simulink model "Racing_2019"  (R2017a)
settings: Solver=FixedStepDiscrete  StartTime=0.0  StopTime=Inf  FixedStep=1e-3  RelTol=1e-3  EnableMultiTasking=on
PostLoadFcn:
  | , if any(exist('dsrtsu_mdlpostloadfcn', 'file') == [2, 3, 6]), try dsrtsu_mdlpostloadfcn('Execute', bdroot); catch fprintf('Error in PostLoadFcn (dsrtsu_mdlpostloadfcn) for model "%s":\n %s\n', bdroot, lasterr); end, end,
undefined symbols (not defined in the file): Accu_Fans_Enable, Accu_Fans_ON, Accu_Fans_PWM, APPS_Bypass, APPS_Value, AUX_Error_Time, Batt_Temp_High_Threshold, Batt_Temp_Low_Threshold, BMS_Error_Time, BMS_Reset, BMS_Reset_Enable, BMS_Status_Bypass, Brake_Plausibility_Threshold, Brake_Threshold, Brakelight_Test, Braking_Torque, BSPD_State_Bypass, Buzzer, Buzzer_Silent, Buzzer_Test, Calibrate, CAN_Rx_FMEA_Enable, CAN_Status_FMEA_Enable, CAN_Tx_FMEA_Enable, Car_Reset, Car_Reset_Enable, Dash_Fan_PWM, DiscIntNeverNeededParam, DRS_Enable, DRS_PWM_OFF, DRS_PWM_ON, ED_Enable, ED_On, Eject_USB, Enable_Kill, Enable_LED_Test, Fans_Left_Enable, Fans_Left_ON, Fans_Left_PWM, Fans_Right_Enable, Fans_Right_ON, Fans_Right_PWM, I_MAX, IGBT_Temp_High_Threshold, IGBT_Temp_Low_Threshold, Inverter_CAN_Tx_Enable, Inverter_Frequency, KW_Max_Regen_Reset, KW_Max_Reset, LV_DCDC_Temp_High_Threshold, LV_DCDC_Temp_Low_Threshold, magnitude, Plausibility_Bypass, Power_Limiter_Killswitch, Power_Target_kW, Pump_Left_Enable, Pump_Left_ON, Pump_Right_Enable, Pump_Right_ON, Pump_Signal_Left ... (+13)
libraries: rtiusbflightreclib x206, simulink x153, rtican x52, powerlib_meascontrol x47, simulink_extras x17, rti1401lib_adc_type4 x6, rti1401lib_dio_type4 x3, rti1401lib_II_base x1
(part 1 of 23)
PreSaveFcn:
  | , if any(exist('dsmpb_private', 'file') == [2, 3, 6]), try, dsmpb_private('dsmpb_mdlclblib', 'PreSave', bdroot); catch, disp(lasterr); end, end,
CloseFcn:
  | , if any(exist('dsmpb_private', 'file') == [2, 3, 6]), try, dsmpb_private('dsmpb_mdlclblib', 'Close', bdroot); catch, disp(lasterr); end, end,
Description:
  | Standard RTI1401 template.
  | Supported Matlab version:  R2017a.
settings Model: Tag=RTI1401  DSRTSU_INTERNAL_RTI_VER=500  DSRTSU_INTERNAL_RTI_TYPE=rti1401  RTICANMMDATA=struct('GeneralSetupData',struct('modelroot',['C:\Users\Vasileios Amoiridis\Documents\dSpaceProjects\R2017a_Racing_2019'],'generalsettings',struct('filesettings',struct('destfolder',struct('Name','RTICANMM_FILES','Check',1),'buildfolder',struct('Name','.','Check',1),'AbsDestfolder',struct('Name',['C:\Users\Vasileios Amoiridis\Documents\dSpaceProjects\R2017a_Racing_2019\RTICANMM_FILES']),'AbsBuildfolder',struct('Name',['C:\Users\Vasileios Amoiridis\Documents\dSpaceProjects\R2017a_Racing_2019']))),'options',struct('addpaths',1,'rmpaths',1,'addtrcexclusion',logical(1),'cannavigator',struct('checkmonitoring',0),'show_usrtrc',0,'use_usrtrc',0),'advanced',struct('options',ones(1,100)),'MPSetup',{{}},'modelname','Racing_2019','block','Racing_2019'))  DSRTSU_INTERNAL_RTIFPGA=90  DSMPB_DATASERVER_ModelPortLibVersion1=8  DSMPB_DATASERVER_DataServerVersion1=6  DSMPB_DATASERVER_DataServerStreamVersion1=3  Creator=Vasileios Amoiridis  LastModifiedBy=Vasileios Amoiridis
settings DataIOCC: SaveOutput=off  SignalLogging=off  DSMLogging=off  SaveTime=off
settings OptimizationCC: BlockReduction=off  ConditionallyExecuteInputs=off  OptimizeBlockIOStorage=off  BufferReuse=off  GlobalBufferReuse=off  ExpressionFolding=off  LocalBlockOutputs=off  LifeSpan=inf
settings DebuggingCC: SFUnexpectedBacktrackingDiag=warning  SFNoUnconditionalDefaultTransitionDiag=warning  SFExecutionAtInitializationDiag=none
settings HardwareCC: ProdBitPerPointer=32  ProdBitPerSizeT=32  ProdBitPerPtrDiffT=32  ProdLargestAtomicInteger=Integer  ProdEndianess=BigEndian  ProdWordSize=32  ProdHWDeviceType=Custom Processor->Custom  TargetIntDivRoundTo=Zero  TargetEndianess=BigEndian  TargetHWDeviceType=Custom Processor->Custom
settings SFSimCC: MATLABDynamicMemAlloc=off
settings RTWCC: SystemTargetFile=rti1401.tlc  MakeCommand=make_rti  TemplateMakefile=rti1401.tmf  Description=dSPACE DS1401 Hardware Platform
settings CodeAppCC: GenerateComments=off  SimulinkBlockComments=off
settings STFCustomTargetCC: ParMdlRefBuildCompliant=on  GRTInterface=off  SystemTargetFile=rti1401.tlc
settings GRTTargetCC: TargetLangStandard=C89/C90 (ANSI)  CompOptLevelCompliant=off  ConcurrentExecutionCompliant=off  CombineOutputUpdateFcns=off  MatFileLogging=off  CPPClassGenCompliant=off  UseToolchainInfoCompliant=off
settings ConfigComp: CovMetricSettings=dswe  CovSaveCumulativeToWorkspaceVar=on

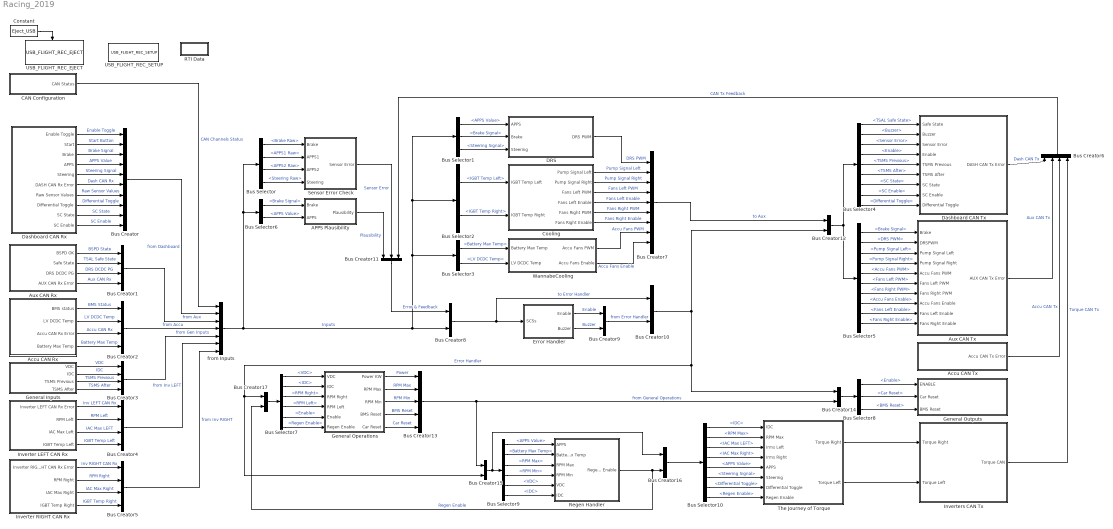
== system Racing_2019 ==
  APPS Plausibility : Subsystem
  Accu CAN Rx : Subsystem
  Accu CAN Tx : Subsystem
  Aux CAN Rx : Subsystem
  Aux CAN Tx : Subsystem
  Bus Creator : BusCreator  Inputs='Enable Toggle','Start Button','Brake Signal','APPS Value','Steering Signal','Dash CAN Rx','Raw Sensor Values','Differential Toggle','SC State','SC Enable'
  Bus Creator1 : BusCreator  Inputs='BSPD State','TSAL Safe State','DRS DCDC PG','Aux CAN Rx'
  Bus Creator{10,12,14..16} (5 alike) : BusCreator  Inputs=2
  Bus Creator11 : BusCreator  Inputs=3
  Bus Creator13 : BusCreator  Inputs=5
  Bus Creator17 : BusCreator  Inputs='Error Handler','Regen Enable'
  Bus Creator2 : BusCreator  Inputs='BMS Status','LV DCDC Temp','Accu CAN Rx','Battery Max Temp'
  Bus Creator3 : BusCreator  Inputs='VDC','IDC','TSMS Previous','TSMS After'
  Bus Creator4 : BusCreator  Inputs='Inv LEFT CAN Rx','RPM Left','IAC Max LEFT','IGBT Temp Left'
  Bus Creator5 : BusCreator  Inputs='Inv RIGHT CAN Rx','RPM Right','IAC Max Right','IGBT Temp Right'
  Bus Creator6 : BusCreator  Inputs='Dash CAN Tx','Aux CAN Tx','Accu CAN Tx','Torque CAN Tx'
  Bus Creator7 : BusCreator  Inputs='DRS PWM','Pump Signal Left','Pump Signal Right','Fans Left PWM','Fans Left Enable','Fans Right PWM','Fans Right Enable','Accu Fans PWM','Accu Fans Enable'
  Bus Creator8 : BusCreator  Inputs='Error & Feedback','Inputs'
  Bus Creator9 : BusCreator  Inputs='Enable','Buzzer'
  Bus Selector : BusSelector  OutputSignals=from Dashboard.Raw Sensor Values.Brake Raw,from Dashboard.Raw Sensor Values.APPS1 Raw,from Dashboard.Raw Sensor Values.APPS2 Raw,from Dashboard.Raw Sensor Values.Steering Raw
  Bus Selector1 : BusSelector  OutputSignals=from Dashboard.APPS Value,from Dashboard.Brake Signal,from Dashboard.Steering Signal
  Bus Selector10 : BusSelector  OutputSignals=signal1.Error Handler.to Error Handler.Inputs.from Gen Inputs.IDC,signal1.from General Operations.RPM Max,signal1.Error Handler.to Error Handler.Inputs.from Inv LEFT.IAC Max LEFT,signal1.Error Handler.to Error Handler.Inputs.from Inv RIGHT.IAC Max Right,signal1.Error Handler.to Error Handler.Inputs.from Dashboard.APPS Value,signal1.Error Handler.to Error Handler.Inputs.from Dashboard.Steering Signal,signal1.Error Handler.to Error Handler.Inputs.from Dashboard.Differential Toggle,Regen Enable
  Bus Selector2 : BusSelector  OutputSignals=from Inv LEFT.IGBT Temp Left,from Inv RIGHT.IGBT Temp Right
  Bus Selector3 : BusSelector  OutputSignals=from Accu.Battery Max Temp,from Accu.LV DCDC Temp
  Bus Selector4 : BusSelector  OutputSignals=Error Handler.to Error Handler.Inputs.from Aux.TSAL Safe State,Error Handler.from Error Handler.Buzzer,Error Handler.to Error Handler.Error & Feedback.Sensor Error,Error Handler.from Error Handler.Enable,Error Handler.to Error Handler.Inputs.from Gen Inputs.TSMS Previous,Error Handler.to Error Handler.Inputs.from Gen Inputs.TSMS After,Error Handler.to Error Handler.Inputs.from Dashboard.SC State,Error Handler.to Error Handler.Inputs.from Dashboard.SC Enable,Error Handler.to Error Handler.Inputs.from Dashboard.Differential Toggle
  Bus Selector5 : BusSelector  OutputSignals=Error Handler.to Error Handler.Inputs.from Dashboard.Brake Signal,to Aux.DRS PWM,to Aux.Pump Signal Left,to Aux.Pump Signal Right,to Aux.Accu Fans PWM,to Aux.Fans Left PWM,to Aux.Fans Right PWM,to Aux.Accu Fans Enable,to Aux.Fans Left Enable,to Aux.Fans Right Enable
  Bus Selector6 : BusSelector  OutputSignals=from Dashboard.Brake Signal,from Dashboard.APPS Value
  Bus Selector7 : BusSelector  OutputSignals=Error Handler.to Error Handler.Inputs.from Gen Inputs.VDC,Error Handler.to Error Handler.Inputs.from Gen Inputs.IDC,Error Handler.to Error Handler.Inputs.from Inv RIGHT.RPM Right,Error Handler.to Error Handler.Inputs.from Inv LEFT.RPM Left,Error Handler.from Error Handler.Enable,Regen Enable
  Bus Selector8 : BusSelector  OutputSignals=Error Handler.from Error Handler.Enable,from General Operations.Car Reset,from General Operations.BMS Reset
  Bus Selector9 : BusSelector  OutputSignals=Error Handler.to Error Handler.Inputs.from Dashboard.APPS Value,Error Handler.to Error Handler.Inputs.from Accu.Battery Max Temp,from General Operations.RPM Max,from General Operations.RPM Min,Error Handler.to Error Handler.Inputs.from Gen Inputs.VDC,Error Handler.to Error Handler.Inputs.from Gen Inputs.IDC
  CAN Configuration : Subsystem
  Constant : Constant  Value=Eject_USB
  Cooling : Subsystem
  DRS : Subsystem
  Dashboard CAN Rx : Subsystem
  Dashboard CAN Tx : Subsystem
  Error Handler : Subsystem
  General Inputs : Subsystem
  General Operations : Subsystem
  "General Outputs " : Subsystem
  Inverter LEFT CAN Rx : Subsystem
  Inverter RIGHT CAN Rx : Subsystem
  Inverters CAN Tx : Subsystem
  RTI Data : Subsystem  Tag=struct('RTIDataServer',struct('RTIDataServerVs','2','RTIModelDescription','struct(''main'',''Racing_2019'',''sub'','''',''isMp'',0)'))  LoadFcn="if exist('rtidc'), try,  rtidc('DataHostBlockClbLoad', gcbh); catch, disp(['Warning: ''LoadFcn'' for RTI Data block failed: ' lasterr]); end, end,"  mask(RTI_DATA_HOST){}
      mask help:
      | RTI Data Block.
      | This block is used by RTI to store internal model-dependent data.
      | Please keep this block on the root level of the model. Deleting this block will result in data loss.
      |
      | NEVER DELETE OR COPY THIS BLOCK!
      settings: CopyFcn="if exist('rtidc'), try,  rtidc('DataHostBlockClbCopy', gcbh); catch, disp(['Warning: ''CopyFcn'' for RTI Data block failed: ' lasterr]); end, end,"  DeleteFcn="if exist('rtidc'), try,  rtidc('DataHostBlockClbDelete', gcbh); catch, disp(['Warning: ''DeleteFcn'' for RTI Data block failed: ' lasterr]); end, end,"  ModelCloseFcn="if exist('rtidc'), try,  rtidc('DataHostBlockClbModelClose', gcbh); catch, disp(['Warning: ''ModelCloseFcn'' for RTI Data block failed: ' lasterr]); end, end,"  PreSaveFcn="if exist('rtidc'), try,  rtidc('DataHostBlockClbPreSave', gcbh); catch, disp(['Warning: ''PreSaveFcn'' for RTI Data block failed: ' lasterr]); end, end,"  PostSaveFcn="if exist('rtidc'), try,  rtidc('DataHostBlockClbPostSave', gcbh); catch, disp(['Warning: ''PostSaveFcn'' for RTI Data block failed: ' lasterr]); end, end,"  NameChangeFcn="if exist('rtidc'), try,  rtidc('DataHostBlockClbNameChange', gcbh); catch, disp(['Warning: ''NameChangeFcn'' for RTI Data block failed: ' lasterr]); end, end,"
      mask Help:
      | RTI Data Block.
      | This block is used by RTI to store internal model-dependent data.
      | Please keep this block on the root level of the model. Deleting this block will result in data loss.
      | 
      | NEVER DELETE OR COPY THIS BLOCK!
      mask Display:
      | text(0.5, 0.5, 'RTI Data', 'HorizontalAlignment', 'center');
      | plot([1 0]);
  Regen Handler : Subsystem
  Sensor Error Check : Subsystem
  The Journey of Torque : Subsystem
  USB_FLIGHT_REC_EJECT : rtiusbflightreclib/USB_FLIGHT_REC_EJECT  DSProperties=struct('RTI',struct('Version',uint32(1),'BlockType',struct('isSLSource',uint8(0),'isSLSink',uint8(1),'isHWSource',uint8(0),'isHWSink',uint8(1),'isSetup',uint8(0),'isInline',uint8(1),'isNonInline',uint8(0),'isInterrupt',uint8(0),'isChannelwise',uint8(1)),'IOBoardType',{{'DSUSB','FLIGHTREC'}},'UnitType','FLIGHTREC','Identifier','EJECT','DialogType','ML','BlockSet','RTIUSBFLIGHTREC','SlaveProcessor','NONE'))  RTIBlockInterface=struct('OutputPortsWidth',int32(1),'OutputPortsActive',0,'TriggerPort',{{'rising'}},'BlockDisplay',{{['USB Flight Recorder\n Eject USB Device'],'center'}},'IconTransparency','on','InitLevel',3,'DialogFcn','rtiusbflightrecejectgui','BlockName',struct('Token',{{'USB_FLIGHT_REC_EJECT'}}))  RTIBlockParameters=struct('TLCFileName',{{'rtiusbflightreceject','OFF',[]}})  RTISFcnParameters=struct('TLCFileName','char')  RTIBlockParaDefault=struct('TLCFileName','rtiusbflightreceject')
      settings: SourceProductName=dSPACE RTI USB Flight Rec Blockset
  USB_FLIGHT_REC_SETUP : rtiusbflightreclib/USB_FLIGHT_REC_SETUP  BufferOverwriteMode=Replace old data  TLCFileName=rtiusbflightrecsetup  DSProperties=struct('RTI',struct('Version',uint32(1),'BlockType',struct('isSLSource',uint8(0),'isSLSink',uint8(0),'isHWSource',uint8(0),'isHWSink',uint8(0),'isSetup',uint8(1),'isInline',uint8(1),'isNonInline',uint8(0),'isInterrupt',uint8(0),'isChannelwise',uint8(0)),'IOBoardType',{{'DSUSB','FLIGHTREC'}},'UnitType','FLIGHTREC','Identifier','SETUP','DialogType','SL','BlockSet','RTIUSBFLIGHTREC','SlaveProcessor','NONE'))  RTIBlockInterface=struct('OutputPortsActive',0,'OutputPortsWidth',int32(1),'BlockDisplay',{{['USB Flight Recorder\n Setup'],'center'}},'IconTransparency','off','InitLevel',3,'BlockName',struct('Token',{{'USB_FLIGHT_REC_SETUP'}}),'MaskDescription',['Initializes the USB device for flight recording.'])  RTIBlockParameters=struct('BufferOverwriteMode',{{2,'OFF',[1 2]}},'TLCFileName',{{'rtiusbflightrecsetup','OFF',[]}})  RTISFcnParameters=struct('BufferOverwriteMode','double','TLCFileName','char')  RTIBlockParaDefault=struct('BufferOverwriteMode',1,'TLCFileName','rtiusbflightrecsetup')
      settings: SourceProductName=dSPACE RTI USB Flight Rec Blockset
  WannabeCooling : Subsystem
  from Inputs : BusCreator  Inputs='CAN Channels Status','from Dashboard','from Aux','from Accu','from Gen Inputs','from Inv LEFT','from Inv RIGHT'
  wires:
  Constant/1 -> USB_FLIGHT_REC_EJECT/Trigger
  Dashboard CAN Rx/1(Enable Toggle) -> Bus Creator/1  "Enable Toggle"
  Dashboard CAN Rx/2(Start) -> Bus Creator/2  "Start Button"
  Dashboard CAN Rx/4(APPS) -> Bus Creator/4  "APPS Value"
  Dashboard CAN Rx/5(Steering) -> Bus Creator/5  "Steering Signal"
  Dashboard CAN Rx/6(DASH CAN Rx Error) -> Bus Creator/6  "Dash CAN Rx"
  Aux CAN Rx/1("BSPD OK ") -> Bus Creator1/1  "BSPD State"
  Aux CAN Rx/2(Safe State) -> Bus Creator1/2  "TSAL Safe State"
  Aux CAN Rx/3(DRS DCDC PG) -> Bus Creator1/3  "DRS DCDC PG"
  Aux CAN Rx/4("AUX CAN Rx Error ") -> Bus Creator1/4  "Aux CAN Rx"
  Accu CAN Rx/1(BMS status) -> Bus Creator2/1  "BMS Status"
  Accu CAN Rx/2(LV DCDC Temp) -> Bus Creator2/2  "LV DCDC Temp"
  Accu CAN Rx/3("Accu CAN Rx Error ") -> Bus Creator2/3  "Accu CAN Rx"
  Accu CAN Rx/4(Battery Max Temp) -> Bus Creator2/4  "Battery Max Temp"
  General Inputs/1(VDC) -> Bus Creator3/1  "VDC"
  General Inputs/2(IDC) -> Bus Creator3/2  "IDC"
  Inverter LEFT CAN Rx/1(Inverter LEFT CAN Rx Error) -> Bus Creator4/1  "Inv LEFT CAN Rx"
  Inverter LEFT CAN Rx/2(RPM Left) -> Bus Creator4/2  "RPM Left"
  Inverter LEFT CAN Rx/3(IAC Max Left) -> Bus Creator4/3  "IAC Max LEFT"
  Inverter LEFT CAN Rx/4(IGBT Temp Left) -> Bus Creator4/4  "IGBT Temp Left"
  Inverter RIGHT CAN Rx/1(Inverter RIGHT CAN Rx Error) -> Bus Creator5/1  "Inv RIGHT CAN Rx"
  Inverter RIGHT CAN Rx/2(RPM Right) -> Bus Creator5/2  "RPM Right"
  Inverter RIGHT CAN Rx/3(IAC Max Right) -> Bus Creator5/3  "IAC Max Right"
  Inverter RIGHT CAN Rx/4(IGBT Temp Right) -> Bus Creator5/4  "IGBT Temp Right"
  CAN Configuration/1(CAN Status) -> from Inputs/1  "CAN Channels Status"
  Bus Creator/1 -> from Inputs/2  "from Dashboard"
  Bus Creator1/1 -> from Inputs/3  "from Aux"
  Bus Creator2/1 -> from Inputs/4  "from Accu"
  Bus Creator3/1 -> from Inputs/5  "from Gen Inputs"
  Bus Creator4/1 -> from Inputs/6  "from Inv LEFT"
  Bus Creator5/1 -> from Inputs/7  "from Inv RIGHT"
  Dashboard CAN Tx/1(DASH CAN Tx Error) -> Bus Creator6/1  "Dash CAN Tx"
  Aux CAN Tx/1(AUX CAN Tx Error) -> Bus Creator6/2  "Aux CAN Tx"
  Accu CAN Tx/1(Accu CAN Tx Error) -> Bus Creator6/3  "Accu CAN Tx"
  Inverters CAN Tx/1("Torque CAN ") -> Bus Creator6/4  "Torque CAN Tx"
  Dashboard CAN Rx/7(Raw Sensor Values) -> Bus Creator/7  "Raw Sensor Values"
  from Inputs/1 -> Bus Selector/1, Bus Selector6/1, Bus Selector1/1, Bus Selector2/1, Bus Selector3/1, Bus Creator8/2  "Inputs"
  Bus Selector/1 -> Sensor Error Check/1("Brake ")  "<Brake Raw>"
  Bus Selector/2 -> Sensor Error Check/2(APPS1)  "<APPS1 Raw>"
  Bus Selector/3 -> Sensor Error Check/3(APPS2)  "<APPS2 Raw>"
  Bus Selector/4 -> Sensor Error Check/4(Steering)  "<Steering Raw>"
  Cooling/2(Pump Signal Right) -> Bus Creator7/3  "Pump Signal Right"
  DRS/1(DRS PWM) -> Bus Creator7/1  "DRS PWM"
  Cooling/1(Pump Signal Left) -> Bus Creator7/2  "Pump Signal Left"
  WannabeCooling/1(Accu Fans PWM) -> Bus Creator7/8  "Accu Fans PWM"
  Cooling/4(Fans Left Enable) -> Bus Creator7/5  "Fans Left Enable"
  Cooling/3("Fans Left PWM ") -> Bus Creator7/4  "Fans Left PWM"
  Cooling/5(Fans Right PWM) -> Bus Creator7/6  "Fans Right PWM"
  WannabeCooling/2(Accu Fans Enable) -> Bus Creator7/9  "Accu Fans Enable"
  Cooling/6(Fans Right Enable) -> Bus Creator7/7  "Fans Right Enable"
  Bus Selector1/1 -> DRS/1("APPS ")  "<APPS Value>"
  Bus Selector1/2 -> DRS/2("Brake ")  "<Brake Signal>"
  Bus Selector1/3 -> DRS/3(Steering)  "<Steering Signal>"
  Bus Selector2/1 -> Cooling/1(IGBT Temp Left)  "<IGBT Temp Left>"
  Bus Selector2/2 -> Cooling/2(IGBT Temp Right)  "<IGBT Temp Right>"
  Bus Selector3/1 -> WannabeCooling/1(Battery Max Temp)  "<Battery Max Temp>"
  Bus Selector3/2 -> WannabeCooling/2(LV DCDC Temp)  "<LV DCDC Temp>"
  Bus Selector5/2 -> Aux CAN Tx/2("DRSPWM ")  "<DRS PWM>"
  Bus Selector5/3 -> Aux CAN Tx/3(Pump Signal Left)  "<Pump Signal Left>"
  Bus Selector5/4 -> Aux CAN Tx/4(Pump Signal Right)  "<Pump Signal Right>"
  Bus Selector5/7 -> Aux CAN Tx/7(Fans Right PWM)  "<Fans Right PWM>"
  Bus Selector5/1 -> Aux CAN Tx/1(Brake)  "<Brake Signal>"
  Sensor Error Check/1(Sensor Error) -> Bus Creator11/2  "Sensor Error"
  Bus Creator6/1 -> Bus Creator11/3  "CAN Tx Feedback"
  Bus Creator8/1 -> Bus Creator10/1, Error Handler/1(SCSs)  "to Error Handler"
  Bus Selector6/1 -> APPS Plausibility/1(Brake)  "<Brake Signal>"
  Bus Selector6/2 -> APPS Plausibility/2(APPS)  "<APPS Value>"
  APPS Plausibility/1(Plausibility) -> Bus Creator11/1  "Plausibility"
  Error Handler/1(Enable) -> Bus Creator9/1  "Enable"
  Error Handler/2(Buzzer) -> Bus Creator9/2  "Buzzer"
  Bus Creator9/1 -> Bus Creator10/2  "from Error Handler"
  Bus Creator11/1 -> Bus Creator8/1  "Error & Feedback"
  Bus Selector4/1 -> Dashboard CAN Tx/1(Safe State)  "<TSAL Safe State>"
  Bus Selector4/2 -> Dashboard CAN Tx/2(Buzzer)  "<Buzzer>"
  Bus Selector4/3 -> Dashboard CAN Tx/3(Sensor Error)  "<Sensor Error>"
  Bus Selector4/4 -> Dashboard CAN Tx/4(Enable)  "<Enable>"
  Bus Creator10/1 -> Bus Creator14/1, Bus Creator17/1, Bus Creator15/2, Bus Creator12/2  "Error Handler"
  Bus Creator7/1 -> Bus Creator12/1  "to Aux"
  Bus Creator12/1 -> Bus Selector5/1, Bus Selector4/1
  Bus Selector5/5 -> Aux CAN Tx/5(Accu Fans PWM)  "<Accu Fans PWM>"
  Bus Selector5/6 -> Aux CAN Tx/6(Fans Left PWM)  "<Fans Left PWM>"
  Bus Selector5/8 -> Aux CAN Tx/8(Accu Fans Enable)  "<Accu Fans Enable>"
  Bus Selector5/9 -> Aux CAN Tx/9(Fans Left Enable)  "<Fans Left Enable>"
  Bus Selector5/10 -> Aux CAN Tx/10(Fans Right Enable)  "<Fans Right Enable>"
  Bus Selector7/1 -> General Operations/1(VDC)  "<VDC>"
  Bus Selector7/2 -> General Operations/2(IDC)  "<IDC>"
  Bus Selector7/3 -> General Operations/3(RPM Right)  "<RPM Right>"
  Bus Selector7/4 -> General Operations/4(RPM Left)  "<RPM Left>"
  Bus Selector7/5 -> General Operations/5(Enable)  "<Enable>"
  General Operations/1(Power KW) -> Bus Creator13/1  "Power"
  General Operations/2(RPM Max) -> Bus Creator13/2  "RPM Max"
  General Operations/3(RPM Min) -> Bus Creator13/3  "RPM Min"
  General Operations/4(BMS Reset) -> Bus Creator13/4  "BMS Reset"
  General Operations/5(Car Reset) -> Bus Creator13/5  "Car Reset"
  Bus Creator13/1 -> Bus Creator15/1, Bus Creator14/2  "from General Operations"
  Bus Creator14/1 -> Bus Selector8/1
  Bus Selector8/1 -> "General Outputs "/1(ENABLE)  "<Enable>"
  Bus Selector8/2 -> "General Outputs "/2(Car Reset)  "<Car Reset>"
  Bus Selector8/3 -> "General Outputs "/3(BMS Reset)  "<BMS Reset>"
  Dashboard CAN Rx/8(Differential Toggle) -> Bus Creator/8  "Differential Toggle"
  Bus Creator15/1 -> Bus Creator16/1, Bus Selector9/1
  Bus Selector9/1 -> Regen Handler/1(APPS)  "<APPS Value>"
  Bus Selector9/2 -> Regen Handler/2(Battery Max Temp)  "<Battery Max Temp>"
  Bus Selector9/3 -> Regen Handler/3(RPM Max)  "<RPM Max>"
  Bus Selector9/4 -> Regen Handler/4(RPM Min)  "<RPM Min>"
  Bus Selector9/5 -> Regen Handler/5(VDC)  "<VDC>"
  Bus Selector9/6 -> Regen Handler/6(IDC)  "<IDC>"
  Regen Handler/1(Regen Enable) -> Bus Creator17/2, Bus Creator16/2  "Regen Enable"
  Bus Creator17/1 -> Bus Selector7/1
  Bus Selector7/6 -> General Operations/6(Regen Enable)  "<Regen Enable>"
  Bus Creator16/1 -> Bus Selector10/1
  Bus Selector10/1 -> The Journey of Torque/1("IDC ")  "<IDC>"
  Bus Selector10/2 -> The Journey of Torque/2(RPM Max)  "<RPM Max>"
  Bus Selector10/3 -> The Journey of Torque/3(Irms Left)  "<IAC Max LEFT>"
  Bus Selector10/4 -> The Journey of Torque/4(Irms Right)  "<IAC Max Right>"
  Bus Selector10/5 -> The Journey of Torque/5(APPS)  "<APPS Value>"
  Bus Selector10/6 -> The Journey of Torque/6(Steering)  "<Steering Signal>"
  Bus Selector10/7 -> The Journey of Torque/7(Differential Toggle)  "<Differential Toggle>"
  Bus Selector10/8 -> The Journey of Torque/8("Regen Enable ")  "<Regen Enable>"
  The Journey of Torque/1("Torque Right ") -> Inverters CAN Tx/1(Torque Right)
  The Journey of Torque/2(Torque Left) -> Inverters CAN Tx/2(Torque Left)
  Dashboard CAN Rx/3(Brake) -> Bus Creator/3  "Brake Signal"
  General Inputs/3(TSMS Previous) -> Bus Creator3/3  "TSMS Previous"
  General Inputs/4(TSMS After) -> Bus Creator3/4  "TSMS After"
  Bus Selector4/5 -> Dashboard CAN Tx/5(TSMS Previous)  "<TSMS Previous>"
  Bus Selector4/6 -> Dashboard CAN Tx/6(TSMS After)  "<TSMS After>"
  Dashboard CAN Rx/9(SC State) -> Bus Creator/9  "SC State"
  Bus Selector4/7 -> Dashboard CAN Tx/7(SC State)  "<SC State>"
  Dashboard CAN Rx/10(SC Enable) -> Bus Creator/10  "SC Enable"
  Bus Selector4/8 -> Dashboard CAN Tx/8(SC Enable)  "<SC Enable>"
  Bus Selector4/9 -> Dashboard CAN Tx/9(Differential Toggle)  "<Differential Toggle>"

== system Racing_2019/APPS Plausibility ==
  Brake : Inport
  APPS : Inport  Port=2
  Add : Sum
  Compare To Constant : simulink/Logic and Bit Operations/Compare To Constant  relop=>=  const=250  OutDataTypeStr=boolean
  Compare To Constant1 : simulink/Logic and Bit Operations/Compare To Constant  relop=<=  const=100  OutDataTypeStr=boolean
  Constant1 : Constant  Value=Brake_Threshold
  Constant2 : Constant  Value=Brake_Plausibility_Threshold
  Logical Operator : Logic  AllPortsSameDT=off  OutDataTypeStr=boolean
  Relational Operator : RelationalOperator  OutDataTypeStr=boolean  RndMeth=Simplest
  Resettable Delay 350ms : Delay  DelayLength=350  ExternalReset=Rising  SampleTime=0.001
      settings: InputPortMap=u0,r5
  S-R Flip-Flop : simulink_extras/Flip Flops/S-R Flip-Flop  initial_condition=0
  Terminator : Terminator
  Plausibility : Outport
  wires:
  APPS/1 -> Compare To Constant1/1, Compare To Constant/1
  Constant2/1 -> Add/2
  Constant1/1 -> Add/1
  Add/1 -> Relational Operator/2
  Brake/1 -> Relational Operator/1
  Logical Operator/1 -> Resettable Delay 350ms/2, Resettable Delay 350ms/1
  Resettable Delay 350ms/1 -> S-R Flip-Flop/1
  Compare To Constant1/1 -> S-R Flip-Flop/2
  Relational Operator/1 -> Logical Operator/1
  Compare To Constant/1 -> Logical Operator/2
  S-R Flip-Flop/2 -> Terminator/1
  S-R Flip-Flop/1 -> Plausibility/1

== system Racing_2019/Accu CAN Rx ==
  note: Error = ?
  note: Error = 1
  Add : Sum
  BMS : Logic  Operator=NOT  AllPortsSameDT=off  OutDataTypeStr=boolean
  BMS_200 : rtican/RTICAN Receive (RX)   Reserved1=[]  Reserved2=[]  Reserved3=[]  Reserved4=[]  SfcnMessage=[]  Msg_Struct=[]  BoardTypeNo=[]  BoardNo=[]  ChannelNo=[]  Parameters=[]  DialogFcn=[]  UnitName=[]  Revision=[]  UnitValues=[]  DSProperties=struct('RTI',struct('Version',uint32(5),'BlockType',struct('isSLSource',uint8(1),'isSLSink',uint8(1),'isHWSource',uint8(0),'isHWSink',uint8(0),'isSetup',uint8(0),'isInline',uint8(1),'isNonInline',uint8(0),'isInterrupt',uint8(0),'isChannelwise',uint8(0)),'IOBoardType','RTICAN','UnitType','MESSAGE','Identifier','RX','DialogType','MSVC','BlockSet','RTICAN','SlaveProcessor','CAN'))  RTIBlockInterface=struct('OutputPortsWidth',int32([1 1 1 1]),'OutputPortsActive',[1 1 1 1],'OutputPortsName',{{'BMS_Status','Idc','LV_DCDC_Temp',['RX status']}},'OutputPortsDataType',{{'SS_UINT8','SS_INT16','SS_UINT8','SS_DOUBLE'}},'OutputPortsLabel',{{'BMS_Status','Idc','LV_DCDC_Temp',''}},'OutputPortsLabelMode','ON','InputPortsWidth',int32(0),'InputPortsActive',0,'DialogFcn','rtican_message_interface_gui','BlockDisplay',{{'','center'}},'IconTransparency','on','ParameterTunableNames',{{}},'InitLevel',3,'BlockName',struct('Token',{{'BMS_200'}}),'SampleTime',{{0.001}},'TriggerPort',{{'none'}},'EnablePort',{{'none'}})  RTIBlockParameters=struct('BoardTypeNo',{{1,'OFF',[]}},'BoardNo',{{2,'ON',[1 16]}},'ChannelNo',{{1,'ON',[1 2]}},'Parameters',{{struct('DataFileSupport',struct('DataFileSelectedMaster',0,'DataFileSelectedLocal',0,'DataFileName',['<no datafile support>|'],'DataFileDate','','SelectedFile',['<no file selected>']),'Options',struct('StatusSelected',1,'TimeSelected',0,'DeltaTimeSelected',0,'BytePortSelected',0,'MessageLengthSelected',0,'TriggerPort',struct('Selected',0,'TriggerType',0),'UserCoding',struct('Selected',0,'InterfaceFile','UserDecodingFile','FcnName','UserDecodeFcn','InportSelected',0,'InportWidth',1,'OutportSelected',0,'OutportWidth',1),'EnablePortSelected',0,'SignalOnPortnameSelected',1,'UseRXService',0),'Message',struct('MsgOnBlocknameSelected',1,'MsgName','BMS_200','MsgIdFormat',0,'MsgId',200,'MsgLength',8,'NumSignals',3,'SampleTime',0.001,'Signal',struct('SgnName',{'BMS_Status','Idc','LV_DCDC_Temp'},'SgnStartBit',{0,8,40},'SgnLength',{8,16,8},'SgnType',{0,0,0},'ModeValue',{-1,-1,-1},'DataType',{0,1,0},'ByteLayout',{1,1,1},'Factor',{1,1,1},'Offset',{0,0,0},'SgnComment',{{''},{''},{''}},'SgnUnit',{'','',''},'Min',{0,0,0},'Max',{255,255,255},'SLDataType',{'SS_UINT8','SS_INT16','SS_UINT8'}),'MsgIdNumFormat',0,'MsgComment',{{''}}),'Version',1.2,'general',struct('isFromLib',0)),'OFF',[]}},'GroupId',{{struct('Group',{{'RTICAN'}},'No',3,'Behavior',{{'NAMECHANGE'}},'BlockType',{{'SINK'}},'NameChangeFlag',0),'OFF',[]}},'SFcnRTICANMessage',{{struct('MsgType','RX','SFcnPortType','Scalar','MsgName','BMS_200','MsgIdFormat','STD','MsgId',200,'MsgLength',8,'NumSignals',3,'SampleTime',0.001,'Signal',struct('SgnName',{'BMS_Status','Idc','LV_DCDC_Temp'},'SgnStartBit',{0,8,40},'SgnLength',{8,16,8},'SgnType',{'standard','standard','standard'},'ModeValue',{-1,-1,-1},'DataType',{['unsigned int'],['signed int'],['unsigned int']},'ByteLayout',{['big endian'],['big endian'],['big endian']},'Factor',{1,1,1},'Offset',{0,0,0},'SLDataType',{'SS_UINT8','SS_INT16','SS_UINT8'}),'StatusSelected','yes','TimeSelected','no','DeltaTimeSelected','no','BytePortSelected','no','MessageLengthSelected','no','TriggerPort',struct('Selected','no','TriggerType',0),'UserCoding',struct('Selected','no','InterfaceFile','UserDecodingFile','FcnName','UserDecodeFcn','InportSelected','no','InportWidth',1,'OutportSelected','no','OutportWidth',1),'EnablePortSelected','no','UseRXService','no','BoardType','DS1','BoardNo',2,'ControllerNo',1),'OFF',[]}},'TLCFileName',{{'rtican_rx_message','OFF',[]}})  RTISFcnParameters=struct('SFcnRTICANMessage','struct','TLCFileName','char')  RTIBlockParaDefault=struct('BoardTypeNo',4302,'BoardNo',1,'ChannelNo',1,'Parameters',struct('DataFileSupport',struct('DataFileSelectedMaster',0,'DataFileSelectedLocal',0,'DataFileName','','DataFileDate','','SelectedFile',['<no file selected>']),'Options',struct('StatusSelected',1,'TimeSelected',1,'DeltaTimeSelected',1,'BytePortSelected',0,'MessageLengthSelected',0,'TriggerPort',struct('Selected',0,'TriggerType','rising'),'UserCoding',struct('Selected',0,'InterfaceFile','UserDecodingFile','FcnName','UserDecodeFcn','InportSelected',0,'InportWidth',1,'OutportSelected',0,'OutportWidth',1),'EnablePortSelected',0,'SignalOnPortnameSelected',1,'UseRXService',0),'Message',struct('MsgOnBlocknameSelected',0,'MsgName',['RX Message'],'MsgIdFormat',0,'MsgId',100,'MsgLength',8,'NumSignals',1,'SampleTime',-1,'Signal',struct('SgnName',['RX signal'],'SgnStartBit',0,'SgnLength',8,'SgnType',0,'ModeValue',-1,'DataType',0,'SLDataType','SS_DOUBLE','ByteLayout',0,'Factor',1,'Offset',0,'Min',0,'Max',255,'SgnComment',{{}},'SgnUnit',''),'MsgIdNumFormat',0,'MsgComment',{{''}}),'Version',1.2,'general',struct('isFromLib',1)),'GroupId',struct('Group',{{'RTICAN'}},'No',1,'Behavior',{{'NAMECHANGE'}},'BlockType',{{'SINK'}},'NameChangeFlag',0),'SFcnRTICANMessage',struct('MsgType','RX','MsgName',['RX Message'],'MsgIdFormat','STD','MsgId',100,'MsgLength',8,'NumSignals',1,'SampleTime',-1,'Signal',struct('SgnName',['RX signal'],'SgnStartBit',0,'SgnLength',8,'SgnType','standard','ModeValue',-1,'DataType',['unsigned int'],'ByteLayout',['little endian'],'SLDataType','SS_DOUBLE','Factor',1,'Offset',0),'StatusSelected','yes','TimeSelected','yes','DeltaTimeSelected','yes','BytePortSelected','no','MessageLengthSelected','no','EnablePortSelected','no','UserCoding',struct('Selected','no','InterfaceFile','UserDecodingFile','FcnName','UserDecodeFcn','InportSelected','no','InportWidth',1,'OutportSelected','no','OutportWidth',1),'TriggerPort',struct('Selected','no','TriggerType','rising'),'UseRXService','no','BoardType','DS4302','BoardNo',1,'ControllerNo',1,'SFcnPortType','Scalar'),'TLCFileName','rtican_rx_message')
      settings: AttributesFormatString=Group Id: RTICAN3\n  SourceProductName=dSPACE RTI CAN Blockset
  BMS_CAN_200 : Delay  DelayLength=2000  InitialCondition=1  ExternalReset=Level
      settings: InputPortMap=u0,r5
  BMS_CAN_200_Counter : Memory  InheritSampleTime=on
  Bus Creator : BusCreator  Inputs=6
  Bus Creator1 : BusCreator  Inputs='CAN Error s2','Max Voltage s2','Min Voltage s2','Voltage Sum s2','Max Temperature s2','Min Temperature s2'
  Bus Creator2 : BusCreator  Inputs='CAN Error s3','Max Voltage s3','Min Voltage s3','Voltage Sum s3','Max Temperature s3','Min Temperature s3'
  Bus Creator3 : BusCreator  Inputs='CAN Error s4','Max Voltage s4','Min Voltage s4','Voltage Sum s4','Max Temperature s4','Min Temperature s4'
  Bus Creator4 : BusCreator  Inputs='CAN Error s5','Max Voltage s5','Min Voltage s5','Voltage Sum s5','Max Temperature s5','Min Temperature s5'
  Bus Creator5 : BusCreator  Inputs='CAN Error s6','Max Voltage s6','Min Voltage s6','Voltage Sum s6','Max Temperature s6','Min Temperature s6'
  Bus Creator6 : BusCreator  Inputs='CAN Error s7','Max Voltage s7','Min Voltage s7','Voltage Sum s7','Max Temperature s7','Min Temperature s7'
  Bus Creator7 : BusCreator  Inputs=7
  Bus Selector : BusSelector  OutputSignals=signal1.Max Voltage s1,signal2.Max Voltage s2,signal3.Max Voltage s3,signal4.Max Voltage s4,signal5.Max Voltage s5,signal6.Max Voltage s6,signal7.Max Voltage s7
  Bus Selector1 : BusSelector  OutputSignals=signal1.Min Voltage s1,signal2.Voltage Sum s2,signal3.Voltage Sum s3,signal4.Voltage Sum s4,signal5.Voltage Sum s5,signal6.Voltage Sum s6,signal7.Voltage Sum s7
  Bus Selector2 : BusSelector  OutputSignals=signal1.Max Temperature s1,signal2.Max Temperature s2,signal3.Max Temperature s3,signal4.Max Temperature s4,signal5.Max Temperature s5,signal6.Max Temperature s6,signal7.Max Temperature s7
  Bus Selector3 : BusSelector  OutputSignals=signal1.Min Voltage s1,signal2.Min Voltage s2,signal3.Min Voltage s3,signal4.Min Voltage s4,signal5.Min Voltage s5,signal6.Min Voltage s6,signal7.Min Voltage s7
  Bus Selector4 : BusSelector  OutputSignals=signal1.Voltage Sum s1,signal2.Voltage Sum s2,signal3.Voltage Sum s3,signal4.Voltage Sum s4,signal5.Voltage Sum s5,signal6.Voltage Sum s6,signal7.Voltage Sum s7
  Bus Selector5 : BusSelector  OutputSignals=signal1.Min Temperature s1,signal2.Min Temperature s2,signal3.Min Temperature s3,signal4.Min Temperature s4,signal5.Min Temperature s5,signal6.Min Temperature s6,signal7.Min Temperature s7
  Bus Selector6 : BusSelector  OutputSignals=signal1.Voltage Sum s1,signal2.Voltage Sum s2,signal3.Voltage Sum s3,signal4.Voltage Sum s4,signal5.Voltage Sum s5,signal6.Voltage Sum s6,signal7.Voltage Sum s7
  Bus Selector7 : BusSelector  OutputSignals=signal1.CAN Error s1,signal2.CAN Error s2,signal3.CAN Error s3,signal4.CAN Error s4,signal5.CAN Error s5,signal6.CAN Error s6,signal7.CAN Error s7
  CAN Segments Rx Error : Logic  Operator=OR  Inputs=8  AllPortsSameDT=off  OutDataTypeStr=boolean
  CAN_ID200 100Hz to 5Hz : RateTransition  OutPortSampleTime=0.2
  Constant2 : Constant  Value=0
  Data Type Conversion : DataTypeConversion  OutDataTypeStr=int16
  Data Type Conversion1 : DataTypeConversion  OutDataTypeStr=uint8
  Data Type Conversion2 : DataTypeConversion  OutDataTypeStr=uint8
  Data Type Conversion3 : DataTypeConversion  OutDataTypeStr=boolean
  Data Type Conversion69 : DataTypeConversion  OutDataTypeStr=int16
  Data Type Conversion7 : DataTypeConversion  OutDataTypeStr=uint8
  Edge Detector : powerlib_meascontrol/Logic/Edge Detector  model=Rising  ic=0  Ts=-1
      settings: SourceProductName=Simscape Power Systems  SourceProductBaseCode=PS
  Gain84 : Gain  Gain=10  OutDataTypeStr=int16
  HV Voltage : Sum  Inputs=+++++++
  Max Battery Voltage : MinMax  Function=max  Inputs=7
  Max Segment Voltage : MinMax  Function=max  Inputs=7
  Max Temperature : MinMax  Function=max  Inputs=7
  Min Battery Voltage : MinMax  Inputs=7
  Min Segment Voltage : MinMax  Inputs=7
  Min Temperature : MinMax  Inputs=7
  Segment 1 : Subsystem
  Segment 2 : Subsystem
  Segment 3 : Subsystem
  Segment 4 : Subsystem
  Segment 5 : Subsystem
  Segment 6 : Subsystem
  Segment 7 : Subsystem
  Terminator{,1,3..6} (6 alike) : Terminator
  USB_BMS_Status : rtiusbflightreclib/USB_FLIGHT_REC_BL1  VarName=BMS_Status  DataType=UInt8  SampleTime=-1  TLCFileName=rtiusbflightrecwrite  Reserved1=[]  Reserved2=[]  Reserved3=[]  Reserved4=[]  DSProperties=struct('RTI',struct('Version',uint32(3),'BlockType',struct('isSLSource',uint8(0),'isSLSink',uint8(1),'isHWSource',uint8(0),'isHWSink',uint8(0),'isSetup',uint8(0),'isInline',uint8(1),'isNonInline',uint8(0),'isInterrupt',uint8(0),'isChannelwise',uint8(0)),'IOBoardType',{{'DSUSB','FLIGHTREC'}},'UnitType','FLIGHTREC','Identifier','WRITE','DialogType','SL','BlockSet','RTIUSBFLIGHTREC','SlaveProcessor','NONE'))  RTIBlockInterface=struct('InputPortsActive',1,'InputPortsWidth',int32(1),'InputPortsDataType',{{'SS_UINT8'}},'BlockDisplay',{{['Write to\nUSB Flight Recorder'],'center'}},'IconTransparency','off','InitLevel',3,'BlockName',struct('Token',{{'USB_FLIGHT_REC_BL1'}}),'MaskDescription',['Write input to the Flight Recorder. Recorded data can be referenced by the specified variable.'],'SampleTime',{{-1}})  RTIBlockParameters=struct('VarName',{{'BMS_Status','OFF',[]}},'DataType',{{'UInt8','OFF',[]}},'SampleTime',{{-1,'OFF',[]}},'TLCFileName',{{'rtiusbflightrecwrite','OFF',[]}})  RTISFcnParameters=struct('VarName','char','DataType','char','SampleTime','double','TLCFileName','char')  RTIBlockParaDefault=struct('VarName','Var1','DataType','Single','SampleTime',-1,'TLCFileName','rtiusbflightrecwrite')
      settings: SourceProductName=dSPACE RTI USB Flight Rec Blockset
  USB_IDC_Accu : rtiusbflightreclib/USB_FLIGHT_REC_BL1  VarName=Idc_Accu_x10  DataType=Int16  SampleTime=-1  TLCFileName=rtiusbflightrecwrite  Reserved1=[]  Reserved2=[]  Reserved3=[]  Reserved4=[]  DSProperties=struct('RTI',struct('Version',uint32(3),'BlockType',struct('isSLSource',uint8(0),'isSLSink',uint8(1),'isHWSource',uint8(0),'isHWSink',uint8(0),'isSetup',uint8(0),'isInline',uint8(1),'isNonInline',uint8(0),'isInterrupt',uint8(0),'isChannelwise',uint8(0)),'IOBoardType',{{'DSUSB','FLIGHTREC'}},'UnitType','FLIGHTREC','Identifier','WRITE','DialogType','SL','BlockSet','RTIUSBFLIGHTREC','SlaveProcessor','NONE'))  RTIBlockInterface=struct('InputPortsActive',1,'InputPortsWidth',int32(1),'InputPortsDataType',{{'SS_INT16'}},'BlockDisplay',{{['Write to\nUSB Flight Recorder'],'center'}},'IconTransparency','off','InitLevel',3,'BlockName',struct('Token',{{'USB_FLIGHT_REC_BL1'}}),'MaskDescription',['Write input to the Flight Recorder. Recorded data can be referenced by the specified variable.'],'SampleTime',{{-1}})  RTIBlockParameters=struct('VarName',{{'Idc_Accu_x10','OFF',[]}},'DataType',{{'Int16','OFF',[]}},'SampleTime',{{-1,'OFF',[]}},'TLCFileName',{{'rtiusbflightrecwrite','OFF',[]}})  RTISFcnParameters=struct('VarName','char','DataType','char','SampleTime','double','TLCFileName','char')  RTIBlockParaDefault=struct('VarName','Var1','DataType','Single','SampleTime',-1,'TLCFileName','rtiusbflightrecwrite')
      settings: SourceProductName=dSPACE RTI USB Flight Rec Blockset
  USB_VDC_BMS : rtiusbflightreclib/USB_FLIGHT_REC_BL1  VarName=VDC_BMS  DataType=Int16  SampleTime=-1  TLCFileName=rtiusbflightrecwrite  Reserved1=[]  Reserved2=[]  Reserved3=[]  Reserved4=[]  DSProperties=struct('RTI',struct('Version',uint32(3),'BlockType',struct('isSLSource',uint8(0),'isSLSink',uint8(1),'isHWSource',uint8(0),'isHWSink',uint8(0),'isSetup',uint8(0),'isInline',uint8(1),'isNonInline',uint8(0),'isInterrupt',uint8(0),'isChannelwise',uint8(0)),'IOBoardType',{{'DSUSB','FLIGHTREC'}},'UnitType','FLIGHTREC','Identifier','WRITE','DialogType','SL','BlockSet','RTIUSBFLIGHTREC','SlaveProcessor','NONE'))  RTIBlockInterface=struct('InputPortsActive',1,'InputPortsWidth',int32(1),'InputPortsDataType',{{'SS_INT16'}},'BlockDisplay',{{['Write to\nUSB Flight Recorder'],'center'}},'IconTransparency','off','InitLevel',3,'BlockName',struct('Token',{{'USB_FLIGHT_REC_BL1'}}),'MaskDescription',['Write input to the Flight Recorder. Recorded data can be referenced by the specified variable.'],'SampleTime',{{-1}})  RTIBlockParameters=struct('VarName',{{'VDC_BMS','OFF',[]}},'DataType',{{'Int16','OFF',[]}},'SampleTime',{{-1,'OFF',[]}},'TLCFileName',{{'rtiusbflightrecwrite','OFF',[]}})  RTISFcnParameters=struct('VarName','char','DataType','char','SampleTime','double','TLCFileName','char')  RTIBlockParaDefault=struct('VarName','Var1','DataType','Single','SampleTime',-1,'TLCFileName','rtiusbflightrecwrite')
      settings: SourceProductName=dSPACE RTI USB Flight Rec Blockset
  BMS status : Outport
  LV DCDC Temp : Outport  Port=2
  "Accu CAN Rx Error " : Outport  Port=3
  Battery Max Temp : Outport  Port=4
  wires:
  Data Type Conversion7/1 -> USB_BMS_Status/1
  Edge Detector/1 -> Data Type Conversion1/1
  BMS_CAN_200_Counter/1 -> Add/2
  Add/1 -> BMS_CAN_200_Counter/1
  Data Type Conversion1/1 -> Add/1
  BMS_200/4 -> BMS_CAN_200/2, Edge Detector/1
  BMS_200/2 -> Data Type Conversion69/1  "Idc"
  Data Type Conversion3/1 -> BMS status/1
  Data Type Conversion69/1 -> Gain84/1
  Gain84/1 -> USB_IDC_Accu/1
  BMS/1 -> Data Type Conversion7/1, Data Type Conversion3/1
  BMS_200/3 -> Data Type Conversion2/1  "LV_DCDC_Temp"
  Data Type Conversion2/1 -> LV DCDC Temp/1
  BMS_200/1 -> BMS/1  "BMS_Status"
  BMS_CAN_200/1 -> CAN_ID200 100Hz to 5Hz/1
  Segment 2/1(CAN Error s2) -> Bus Creator1/1  "CAN Error s2"
  Segment 2/2(Max Voltage s2) -> Bus Creator1/2  "Max Voltage s2"
  Segment 2/3(Min Voltage s2) -> Bus Creator1/3  "Min Voltage s2"
  Segment 2/4(Voltage Sum s2) -> Bus Creator1/4  "Voltage Sum s2"
  Segment 2/5(Max Temperature s2) -> Bus Creator1/5  "Max Temperature s2"
  Segment 2/6(Min Temperature s2) -> Bus Creator1/6  "Min Temperature s2"
  Segment 3/1(CAN Error s3) -> Bus Creator2/1  "CAN Error s3"
  Segment 3/2(Max Voltage s3) -> Bus Creator2/2  "Max Voltage s3"
  Segment 3/3(Min Voltage s3) -> Bus Creator2/3  "Min Voltage s3"
  Segment 3/4(Voltage Sum s3) -> Bus Creator2/4  "Voltage Sum s3"
  Segment 3/5(Max Temperature s3) -> Bus Creator2/5  "Max Temperature s3"
  Segment 3/6(Min Temperature s3) -> Bus Creator2/6  "Min Temperature s3"
  Segment 4/1(CAN Error s4) -> Bus Creator3/1  "CAN Error s4"
  Segment 4/2(Max Voltage s4) -> Bus Creator3/2  "Max Voltage s4"
  Segment 4/3(Min Voltage s4) -> Bus Creator3/3  "Min Voltage s4"
  Segment 4/4(Voltage Sum s4) -> Bus Creator3/4  "Voltage Sum s4"
  Segment 4/5(Max Temperature s4) -> Bus Creator3/5  "Max Temperature s4"
  Segment 4/6(Min Temperature s4) -> Bus Creator3/6  "Min Temperature s4"
  Segment 5/1(CAN Error s5) -> Bus Creator4/1  "CAN Error s5"
  Segment 5/2(Max Voltage s5) -> Bus Creator4/2  "Max Voltage s5"
  Segment 5/3(Min Voltage s5) -> Bus Creator4/3  "Min Voltage s5"
  Segment 5/4(Voltage Sum s5) -> Bus Creator4/4  "Voltage Sum s5"
  Segment 5/5(Max Temperature s5) -> Bus Creator4/5  "Max Temperature s5"
  Segment 5/6(Min Temperature s5) -> Bus Creator4/6  "Min Temperature s5"
  Segment 6/1(CAN Error s6) -> Bus Creator5/1  "CAN Error s6"
  Segment 6/2(Max Voltage s6) -> Bus Creator5/2  "Max Voltage s6"
  Segment 6/3(Min Voltage s6) -> Bus Creator5/3  "Min Voltage s6"
  Segment 6/4(Voltage Sum s6) -> Bus Creator5/4  "Voltage Sum s6"
  Segment 6/5(Max Temperature s6) -> Bus Creator5/5  "Max Temperature s6"
  Segment 6/6(Min Temperature s6) -> Bus Creator5/6  "Min Temperature s6"
  Segment 7/1(CAN Error s7) -> Bus Creator6/1  "CAN Error s7"
  Segment 7/2(Max Voltage s7) -> Bus Creator6/2  "Max Voltage s7"
  Segment 7/3(Min Voltage s7) -> Bus Creator6/3  "Min Voltage s7"
  Segment 7/4(Voltage Sum s7) -> Bus Creator6/4  "Voltage Sum s7"
  Segment 7/5(Max Temperature s7) -> Bus Creator6/5  "Max Temperature s7"
  Segment 7/6(Min Temperature s7) -> Bus Creator6/6  "Min Temperature s7"
  Bus Creator/1 -> Bus Creator7/1
  Bus Creator1/1 -> Bus Creator7/2
  Bus Creator2/1 -> Bus Creator7/3
  Bus Creator3/1 -> Bus Creator7/4
  Bus Creator4/1 -> Bus Creator7/5
  Bus Creator5/1 -> Bus Creator7/6
  Bus Creator6/1 -> Bus Creator7/7
  Bus Selector/1 -> Max Battery Voltage/1  "<Max Voltage s1>"
  Bus Selector/2 -> Max Battery Voltage/2  "<Max Voltage s2>"
  Bus Selector/3 -> Max Battery Voltage/3  "<Max Voltage s3>"
  Bus Selector/4 -> Max Battery Voltage/4  "<Max Voltage s4>"
  Bus Selector/5 -> Max Battery Voltage/5  "<Max Voltage s5>"
  Bus Selector/6 -> Max Battery Voltage/6  "<Max Voltage s6>"
  Bus Selector/7 -> Max Battery Voltage/7  "<Max Voltage s7>"
  Bus Creator7/1 -> Bus Selector5/1, Bus Selector7/1, Bus Selector6/1, Bus Selector4/1, Bus Selector2/1, Bus Selector1/1, Bus Selector/1, Bus Selector3/1
  Bus Selector2/1 -> Max Temperature/1  "<Max Temperature s1>"
  Bus Selector1/1 -> Max Segment Voltage/1  "<Min Voltage s1>"
  Bus Selector5/1 -> Min Temperature/1  "<Min Temperature s1>"
  Bus Selector3/1 -> Min Battery Voltage/1  "<Min Voltage s1>"
  Bus Selector1/2 -> Max Segment Voltage/2  "<Voltage Sum s2>"
  Bus Selector1/3 -> Max Segment Voltage/3  "<Voltage Sum s3>"
  Bus Selector1/4 -> Max Segment Voltage/4  "<Voltage Sum s4>"
  Bus Selector1/5 -> Max Segment Voltage/5  "<Voltage Sum s5>"
  Bus Selector1/6 -> Max Segment Voltage/6  "<Voltage Sum s6>"
  Bus Selector1/7 -> Max Segment Voltage/7  "<Voltage Sum s7>"
  Bus Selector2/2 -> Max Temperature/2  "<Max Temperature s2>"
  Bus Selector2/3 -> Max Temperature/3  "<Max Temperature s3>"
  Bus Selector2/4 -> Max Temperature/4  "<Max Temperature s4>"
  Bus Selector2/5 -> Max Temperature/5  "<Max Temperature s5>"
  Bus Selector2/6 -> Max Temperature/6  "<Max Temperature s6>"
  Bus Selector2/7 -> Max Temperature/7  "<Max Temperature s7>"
  Bus Selector3/2 -> Min Battery Voltage/2  "<Min Voltage s2>"
  Bus Selector3/3 -> Min Battery Voltage/3  "<Min Voltage s3>"
  Bus Selector3/4 -> Min Battery Voltage/4  "<Min Voltage s4>"
  Bus Selector3/5 -> Min Battery Voltage/5  "<Min Voltage s5>"
  Bus Selector3/6 -> Min Battery Voltage/6  "<Min Voltage s6>"
  Bus Selector3/7 -> Min Battery Voltage/7  "<Min Voltage s7>"
  Bus Selector4/2 -> Min Segment Voltage/2  "<Voltage Sum s2>"
  Bus Selector4/3 -> Min Segment Voltage/3  "<Voltage Sum s3>"
  Bus Selector4/4 -> Min Segment Voltage/4  "<Voltage Sum s4>"
  Bus Selector4/5 -> Min Segment Voltage/5  "<Voltage Sum s5>"
  Bus Selector4/6 -> Min Segment Voltage/6  "<Voltage Sum s6>"
  Bus Selector4/7 -> Min Segment Voltage/7  "<Voltage Sum s7>"
  Bus Selector5/2 -> Min Temperature/2  "<Min Temperature s2>"
  Bus Selector5/3 -> Min Temperature/3  "<Min Temperature s3>"
  Bus Selector5/4 -> Min Temperature/4  "<Min Temperature s4>"
  Bus Selector5/5 -> Min Temperature/5  "<Min Temperature s5>"
  Bus Selector5/6 -> Min Temperature/6  "<Min Temperature s6>"
  Bus Selector5/7 -> Min Temperature/7  "<Min Temperature s7>"
  Bus Selector6/2 -> HV Voltage/2  "<Voltage Sum s2>"
  Bus Selector6/3 -> HV Voltage/3  "<Voltage Sum s3>"
  Bus Selector6/4 -> HV Voltage/4  "<Voltage Sum s4>"
  Bus Selector6/5 -> HV Voltage/5  "<Voltage Sum s5>"
  Bus Selector6/6 -> HV Voltage/6  "<Voltage Sum s6>"
  Bus Selector6/7 -> HV Voltage/7  "<Voltage Sum s7>"
  Bus Selector7/1 -> CAN Segments Rx Error/1  "<CAN Error s1>"
  Bus Selector7/2 -> CAN Segments Rx Error/2  "<CAN Error s2>"
  Bus Selector7/3 -> CAN Segments Rx Error/3  "<CAN Error s3>"
  Bus Selector7/4 -> CAN Segments Rx Error/4  "<CAN Error s4>"
  Bus Selector7/5 -> CAN Segments Rx Error/5  "<CAN Error s5>"
  Bus Selector7/6 -> CAN Segments Rx Error/6  "<CAN Error s6>"
  Bus Selector7/7 -> CAN Segments Rx Error/7  "<CAN Error s7>"
  Max Battery Voltage/1 -> Terminator/1
  Max Segment Voltage/1 -> Terminator1/1
  Max Temperature/1 -> Battery Max Temp/1
  Min Battery Voltage/1 -> Terminator3/1
  Min Segment Voltage/1 -> Terminator4/1
  Min Temperature/1 -> Terminator5/1
  HV Voltage/1 -> Data Type Conversion/1, Terminator6/1
  CAN Segments Rx Error/1 -> "Accu CAN Rx Error "/1
  Segment 1/1(CAN Error s1) -> Bus Creator/1  "CAN Error s1"
  Segment 1/2(Max Voltage s1) -> Bus Creator/2  "Max Voltage s1"
  Segment 1/3(Min Voltage s1) -> Bus Creator/3  "Min Voltage s1"
  Segment 1/4(Voltage Sum s1) -> Bus Creator/4  "Voltage Sum s1"
  Segment 1/5(Max Temperature s1) -> Bus Creator/5  "Max Temperature s1"
  Segment 1/6(Min Temperature s1) -> Bus Creator/6  "Min Temperature s1"
  CAN_ID200 100Hz to 5Hz/1 -> CAN Segments Rx Error/8
  Bus Selector6/1 -> HV Voltage/1  "<Voltage Sum s1>"
  Bus Selector4/1 -> Min Segment Voltage/1  "<Voltage Sum s1>"
  Constant2/1 -> BMS_CAN_200/1
  Data Type Conversion/1 -> USB_VDC_BMS/1
